simulink model "d_hvdc"  (Simulink 5.1)
settings: Solver=ode45  StartTime=0.0  StopTime=10.0  RelTol=1e-3
libraries: fm_lib x5
settings Model: Creator=fmilano  LastModifiedBy=fmilano  ExtModeAutoUpdateStatusClock=off  SignalLoggingName=logsout  RTWOptions="-aEnforceIntegerDowncast=1 -aFoldNonRolledExpr=1 -aInlineInvariantSignals=1 -aInlineParameters=0 -aLocalBlockOutputs=1 -aRollThreshold=5 -aZeroInternalMemoryAtStartup=1 -aZeroExternalMemoryAtStartup=1 -aInitFltsAndDblsToZero=1 -aForceBlockIOInitOptimize=0 -aGenerateReport=0 -aGenCodeOnly=0 -aRTWVerbose=1 -aIncludeHyperlinkInReport=0 -aLaunchReport=0 -aGenerateTraceInfo=0  -aForceParamTrailComments=0 -aGenerateComments=1 -aIgnoreCustomStorageClasses=1 -aIncHierarchyInIds=0 -aMaxRTWIdLen=31 -aShowEliminatedStatements=0 -aIncDataTypeInIds=0 -aInsertBlockDesc=0 -aIgnoreTestpoints=0 -aSimulinkBlockComments=1 -aInlinedPrmAccess=\"Literals\"  -aSuppressErrorStatus=0 -aModelReferenceCompliant=1 -aParenthesesLevel=\"Nominal\" -aModelStepFunctionPrototypeControlCompliant=0 -aPortableWordSizes=0 -aParMdlRefBuildCompliant=1 -aSupportNonInlinedSFcns=1 -aSupportContinuousTime=1 -aSupportComplex=1 -aSupportNonFinite=1 -aSupportAbsoluteTime=1 -aMultiwordLength=2048 -aTargetPreCompLibLocation=\"\" -aTargetLibSuffix=\"\" -aTargetFunctionLibrary=\"ANSI_C\" -aTargetFcnLib=\"ansi_tfl_tmw.mat\" -aMultiInstanceERTCode=0 -aLogVarNameModifier=\"rt_\" -aERTFirstTimeCompliant=0 -aIsPILTarget=0 -aCombineOutputUpdateFcns=0 -aGenerateASAP2=0 -aGenerateClassInterface=0 -aGenerateTestInterfaces=0 -aGenerateSampleERTMain=0 -aGenerateFullHeader=1 -aUtilityFuncGeneration=\"Auto\" -aIncludeFileDelimiter=\"Auto\" -aIncludeMdlTerminateFcn=1 -aPurelyIntegerCode=0 -aAutosarCompliant=0 -aERTCustomFileBanners=0 -aRTWCAPIStates=0 -aRTWCAPIParams=0 -aRTWCAPISignals=0 -aMatFileLogging=1 -aCompOptLevelCompliant=0 -aCPPClassGenCompliant=0 -aExtModeIntrfLevel=\"Level1\" -aExtModeMexFile=\"ext_comm\" -aExtModeTransport=0 -aExtModeStaticAllocSize=1000000 -aExtModeTesting=0 -aExtModeStaticAlloc=0 -aExtMode=0 -aERTMultiwordLength=256 -aERTMultiwordTypeDef=\"System defined\"  -aGenerateTraceInfo=0 -aGenerateTraceInfo=0 -aGenerateTraceInfo=0 -aGenerateTraceInfo=0 -aPrefixModelToSubsysFcnNames=1"

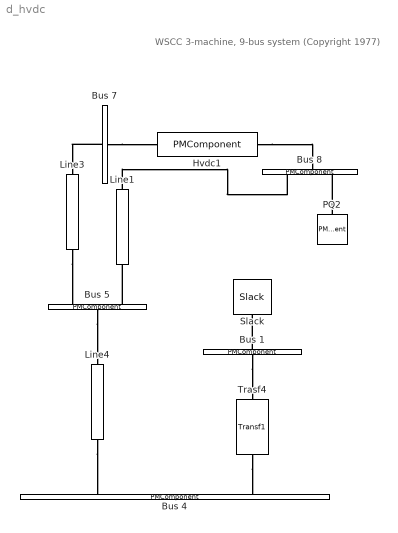
== system d_hvdc ==
  note: WSCC 3-machine, 9-bus system (Copyright 1977)
  Bus 1 : PMComponent  Tag=PSATblock  Description=Connection  Orientation=down  PhysicalDomain=psatdomain  LeftPortType=p1  RightPortType=p1  LConnTagsString=__newl0  RConnTagsString=__newr0  mask(Bus){in=1, out=1, p2q=16.5, p3_4q=[1.00   0.00], p5q=4, p6q=1}
      mask prompts: in "Number of inputs:"; out "Number of outputs:"; p2q "Voltage Rating [kV]"; p3_4q "Voltage initial guess [p.u.  rad]"; p5q "Area number"; p6q "Region number"
      mask help: Bus block.
      mask init:
      | fm_inout
      mask CallbackString: ||||fm_block|
      mask Display: plot([0 1 1 0 0],[0 0 1 1 0])
  Bus 4 : PMComponent  Tag=PSATblock  Description=Connection  Orientation=down  PhysicalDomain=psatdomain  LeftPortType=p1  RightPortType=p1  LConnTagsString=__newl0|__newl1  mask(Bus){in=2, out=0, p2q=230, p3_4q=[1.00   0.00], p5q=2, p6q=1}
      mask prompts: in "Number of inputs:"; out "Number of outputs:"; p2q "Voltage Rating [kV]"; p3_4q "Voltage initial guess [p.u.  rad]"; p5q "Area number"; p6q "Region number"
      mask help: Bus block.
      mask init:
      | fm_inout
      mask CallbackString: ||||fm_block|
      mask Display: plot([0 1 1 0 0],[0 0 1 1 0])
  Bus 5 : PMComponent  Tag=PSATblock  Description=Connection  Orientation=down  PhysicalDomain=psatdomain  LeftPortType=p1  RightPortType=p1  LConnTagsString=__newl0|__newl1  RConnTagsString=__newr0  mask(Bus){in=2, out=1, p2q=230, p3_4q=[1.00   0.00], p5q=2, p6q=1}
      mask prompts: in "Number of inputs:"; out "Number of outputs:"; p2q "Voltage Rating [kV]"; p3_4q "Voltage initial guess [p.u.  rad]"; p5q "Area number"; p6q "Region number"
      mask help: Bus block.
      mask init:
      | fm_inout
      mask CallbackString: ||||fm_block|
      mask Display: plot([0 1 1 0 0],[0 0 1 1 0])
  Bus 7 : PMComponent  Tag=PSATblock  Description=Connection  PhysicalDomain=psatdomain  LeftPortType=p1  RightPortType=p1  LConnTagsString=__newl0  RConnTagsString=__newr0  mask(Bus){in=1, out=1, p2q=230, p3_4q=[1.00   0.00], p5q=2, p6q=1}
      mask prompts: in "Number of inputs:"; out "Number of outputs:"; p2q "Voltage Rating [kV]"; p3_4q "Voltage initial guess [p.u.  rad]"; p5q "Area number"; p6q "Region number"
      mask help: Bus block.
      mask init:
      | fm_inout
      mask CallbackString: ||||fm_block|
      mask Display: plot([0 1 1 0 0],[0 0 1 1 0])
  Bus 8 : PMComponent  Tag=PSATblock  Description=Connection  Orientation=down  PhysicalDomain=psatdomain  LeftPortType=p1  RightPortType=p1  LConnTagsString=__newl0  RConnTagsString=__newr0|__newr1  mask(Bus){in=1, out=2, p2q=230, p3_4q=[1.00   0.00], p5q=2, p6q=1}
      mask prompts: in "Number of inputs:"; out "Number of outputs:"; p2q "Voltage Rating [kV]"; p3_4q "Voltage initial guess [p.u.  rad]"; p5q "Area number"; p6q "Region number"
      mask help: Bus block.
      mask init:
      | fm_inout
      mask CallbackString: ||||fm_block|
      mask Display: plot([0 1 1 0 0],[0 0 1 1 0])
  Hvdc1 : PMComponent  Tag=PSATblock  Description=FACTS  PhysicalDomain=psatdomain  LeftPortType=p1  RightPortType=p1  LConnTagsString=__newl0  RConnTagsString=__newr0  mask(Hvdc){p3_6q=[100  60], p4_5q=[230 230], p7_8q=[300 0.3], p9_10q=[0.1345   0.1257], p11_12q=[1.25  1.25], p13_14q=[20  25], p15_16q=[0.0625  0.200], p17_18q=[120  5], p19_20q=[40  18], p21_22_23_24q=[1.0   0.1  0.9  0.0], p25q=Current_control, p26_27_28q=[0.5  0.5  1.1], p29q=on}
      mask prompts: p3_6q "Power and Frequency Ratings [MVA,  Hz]"; p4_5q "Voltage Rating at Terminal Buses [kV, kV]"; p7_8q "DC Ratings (Vn_dc, In_dc) [kV, kA]"; p9_10q "Transformer Reactances (Xcr  Xci) [p.u.  p.u.]"; p11_12q "Tap Ratios (Ar Ai) [p.u./p.u.  p.u./p.u.]"; p13_14q "PI Regulator Constants (Ki, Kp)"; p15_16q "DC Line Parameters (Rdc Ldc) [p.u.  p.u.]"; p17_18q "Rectifier Angle Limits (a_max, a_min) [deg  deg]"; p19_20q "Inverter Angle Limits (g_max, g_min) [deg  deg]"; p21_22_23_24q "Reference dc current limits (Ir_max, Ir_min, Ii_max, Ii_min) [p.u.]"; p25q "Control type"; p26_27_28q "Current, active power and dc voltage orders [p.u.  p.u.  p.u.]"; p29q "Connected"
      mask help: This block defines a HVDC connection.
      mask init:
      | [x,y] = fm_draw('circle');
      mask StyleString: edit,edit,edit,edit,edit,edit,edit,edit,edit,edit,popup(Current_control|Power_control|Voltage_control),edit,checkbox
      mask CallbackString: ||||||||||||fm_block
      mask Display:
      | plot(0.7+[0 4 4 0 0],[-2 -2 2 2 -2])
      | plot(9.7+[0 4 4 0 0],[-2 -2 2 2 -2])
      | plot([4.7 9.7],[-1.25 -1.25],[4.7 9.7],[1.25 1.25])
      | 
      | plot(x-2,y,x-0.6,y,x+15,y,x+16.4,y)
      | color('green')
      | plot(-2+[-1 -1.3],[0 0],-2+[2.4 2.7],[0 0])
      | plot(-2+[-0.8 0.7],[-1.2 1.2],-2+[0.5 0.7],[1.1 1.2],-2+[0.7 0.7],[1.0 1.2])
      | plot(15+[-1 -1.3],[0 0],15+[2.4 2.7],[0 0])
      | plot(16.4+[-0.8 0.7],[-1.2 1.2],16.4+[0.5 0.7],[1.1 1.2],16.4+[0.7 0.7],[1.0 1.2])
      | 
      | color('magenta')
      | text(1.1,1.2,'R')
      | text(10.1,1.2,'I')
      | plot(0.7+[1 3 2 1],[-0.9 -0.9 0.9 -0.9])
      | plot(9.7+[1 3 2 1],[-0.9 -0.9 0.9 -0.9])
      | plot(0.7+[2 2],[0.9 1.25],0.7+[2 2],[-0.9 -1.25],0.7+[1.2 2.8],[0.9 0.9])
      | plot(9.7+[2 2],[0.9 1.25],9.7+[2 2],[-0.9 -1.25],9.7+[1.2 2.8],[0.9 0.9])
      | plot(0.7+[2 2.5],[0.9 1.25],9.7+[2 2.5],[0.9 1.25])
  Line1 : fm_lib/Power Flow/Line  Tag=PSATblock  Description=Power Flow  Orientation=down  PhysicalDomain=psatdomain  SubClassName=unknown  LeftPortType=p1  RightPortType=p1  LConnTagsString=__newl0  RConnTagsString=__newr0  p3_4_5q="[100  230  60]"  p6q=0  p8q=0.032  p9q=0.161  p10q=0.153*2  p13_14_15q="[0.0  0.0  0.0]"  p16q=on
  Line3 : fm_lib/Power Flow/Line  Tag=PSATblock  Description=Power Flow  Orientation=down  PhysicalDomain=psatdomain  SubClassName=unknown  LeftPortType=p1  RightPortType=p1  LConnTagsString=__newl0  RConnTagsString=__newr0  p3_4_5q="[100  230  60]"  p6q=0  p8q=0.032  p9q=0.161  p10q=0.153*2  p13_14_15q="[0.0  0.0  0.0]"  p16q=on
  Line4 : fm_lib/Power Flow/Line  Tag=PSATblock  Description=Power Flow  Orientation=down  PhysicalDomain=psatdomain  SubClassName=unknown  LeftPortType=p1  RightPortType=p1  LConnTagsString=__newl0  RConnTagsString=__newr0  p3_4_5q="[100  230  60]"  p6q=0  p8q=0.01  p9q=0.085  p10q=0.088*2  p13_14_15q="[0.0  0.0  0.0]"  p16q=on
  PQ2 : PMComponent  Tag=PSATblock  Description=Power Flow  Orientation=down  PhysicalDomain=psatdomain  LeftPortType=p1  RightPortType=p1  LConnTagsString=__newl0  mask(PQ){p2_3q=[100  230], p4_5q=[0.50  0.5], p6_7q=[1.2  0.8], p8q=off, p9q=on}
      mask prompts: p2_3q "Power and Voltage Ratings [MVA, kV]"; p4_5q "Active and Reactive Powers [p.u.  p.u.]"; p6_7q "Maximum and Minimum Allowable Voltage [p.u.   p.u.]"; p8q "Allow conversion to impendance for min & max voltage"; p9q "Connected"
      mask help:
      | This block defines a constant power load:
      |
      | P = Pcost.
      | Q = Qcost.
      mask CallbackString: |||fm_block|fm_block
      mask Display: plot([1 -0.5 -0.5 1],[0 0.866 -0.866 0])
  Slack : fm_lib/Power Flow/Slack  Tag=PSATblock  Description=Power Flow  Orientation=down  PhysicalDomain=psatdomain  SubClassName=unknown  LeftPortType=p1  RightPortType=p1  RConnTagsString=__newr0  p2_3q="[100  16.5]"  p4q=1.04  p5q=0.00  p6_7q=[99 -99]  p8_9q="[1.1  0.9]"  p10q=0.80  p11q=1  p12q=on  p13q=on
  Trasf4 : fm_lib/Power Flow/Transf1  Tag=PSATblock  Description=Power Flow  Orientation=down  PhysicalDomain=psatdomain  SubClassName=unknown  LeftPortType=p1  RightPortType=p1  LConnTagsString=__newl0  RConnTagsString=__newr0  p3_4_5q="[100  16.5  60]"  p7q=16.5/230  p8q=0.0  p9q=0.0576  p13_14_15q="[0.0  0.0  0.0]"  p16q=on
  connections:
  Bus 7/LConn1 -- Line3/LConn1
  Bus 1/RConn1 -- Trasf4/LConn1
  Trasf4/RConn1 -- Bus 4/LConn2
  Line4/RConn1 -- Bus 4/LConn1
  Bus 5/RConn1 -- Line4/LConn1
  Line3/RConn1 -- Bus 5/LConn1
  Bus 7/RConn1 -- Hvdc1/LConn1
  Bus 1/LConn1 -- Slack/RConn1
  Hvdc1/RConn1 -- Bus 8/LConn1
  Bus 5/LConn2 -- Line1/RConn1
  PQ2/LConn1 -- Bus 8/RConn2
  Line1/LConn1 -- Bus 8/RConn1
